simulink model "ROO"  (R2025b)
settings: Solver=VariableStepAuto  StartTime=0.0  StopTime=10  FixedStep=1e-4  RelTol=1e-3
values from neighbouring files (symbols this model uses):
  A_new = T * A * T'    [ROO_code.m]
  Ahat = Abb - Ke * Aab    [ROO_code.m]
  B_new = T * B    [ROO_code.m]
  Bhat = (Abb - Ke*Aab)*Ke + Aba - Ke*Aaa    [ROO_code.m]
  C_new = C * T'    [ROO_code.m]
  Chat = [0 0 0 0 ... (first row only)    [ROO_code.m]
  Dhat = [eye(2);            Ke]    [ROO_code.m]
  eta0_observer = double(xu_start_guess - Ke * y_start_guess)    [ROO_code.m]
  fc = 2 * pi * 15    (= 94.2477796077)    [FSO_code.m]    (also in ROO_code.m)
  Fhat = Bb - Ke * Ba    [ROO_code.m]
  K_new = K * T'    [ROO_code.m]
  params =     [model_data.mat]
  x0_plant = [deg2rad(10); 0; 0; 0; 0; 0]    [ROO_code.m]
libraries: simulink_extras x2, commchan3 x1
settings Model: Creator=Lenovo  LastModifiedBy=Lenovo

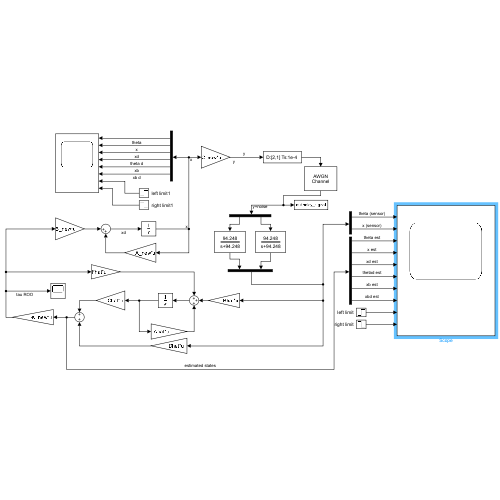
[thumbnail: Simulink's stored preview of the top-level diagram]
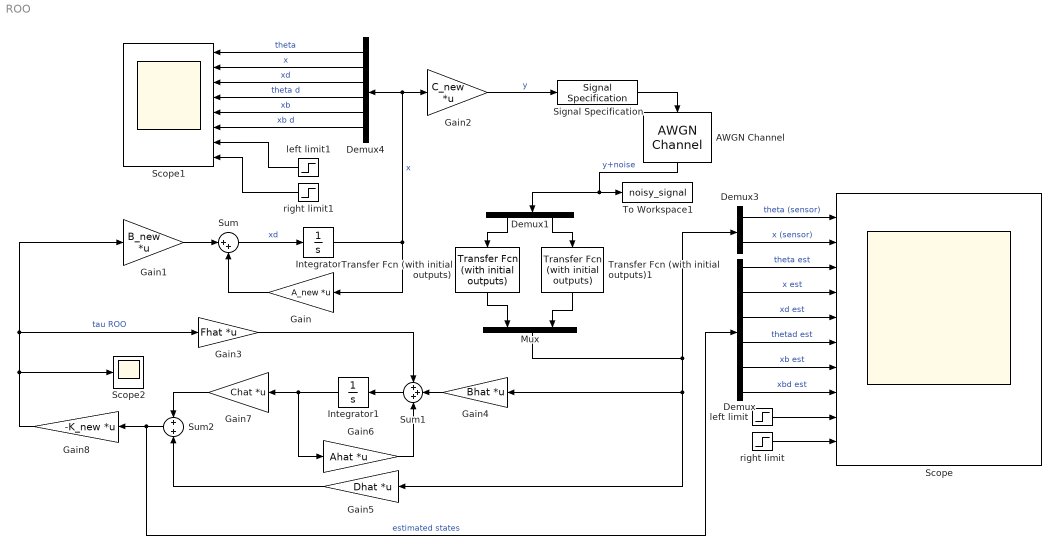
== system ROO ==
  AWGN Channel : commchan3/AWGN Channel  LegacyMode=off  NoiseMethod="Signal to noise ratio  (SNR)"  noiseMode="Signal to noise ratio  (SNR)"  EbNo=10  EsNo=10  SNR=30  BitsPerSymbol=1  SignalPower=1  SpecifySymbolPeriod=off  SamplesPerSymbol=1  SymbolPeriod=1  VarianceSource=Parameter  Variance=1  RandomStream=Global stream  Seed=67  SimulateUsing=Code generation
  Demux : Demux  Outputs=6
  Demux1 : Demux  Outputs=2
  Demux3 : Demux  Outputs=2
  Demux4 : Demux  Outputs=6
  Gain : Gain  Gain=A_new  Multiplication=Matrix(K*u)
  Gain1 : Gain  Gain=B_new  Multiplication=Matrix(K*u)
  Gain2 : Gain  Gain=C_new  Multiplication=Matrix(K*u)
  Gain3 : Gain  Gain=Fhat  Multiplication=Matrix(K*u)
  Gain4 : Gain  Gain=Bhat  Multiplication=Matrix(K*u)
  Gain5 : Gain  Gain=Dhat  Multiplication=Matrix(K*u)
  Gain6 : Gain  Gain=Ahat  Multiplication=Matrix(K*u)
  Gain7 : Gain  Gain=Chat  Multiplication=Matrix(K*u)
  Gain8 : Gain  Gain=-K_new  Multiplication=Matrix(K*u)
  Integrator : Integrator  InitialCondition=x0_plant
  Integrator1 : Integrator  InitialCondition=eta0_observer
  Mux : Mux  Inputs=2
  Scope : Scope  NumInputPorts=10
      settings: SampleTime=1e-4  ActiveDisplayYMinimum=-0.13756249999999998  ActiveDisplayYMaximum=0.13756249999999998
  Scope1 : Scope  NumInputPorts=8
      settings: SampleTime=1e-4  ActiveDisplayYMinimum=-1.4770196744497439  ActiveDisplayYMaximum=11.337524918716566
  Scope2 : Scope
      settings: ActiveDisplayYMinimum=-5.0707763881574976  ActiveDisplayYMaximum=15.205716333962702  DataLoggingVariableName=ScopeData2
  Signal Specification : SignalSpecification  Dimensions=[2,1]  SampleTime=1e-4
  Sum : Sum  Inputs=|++
  Sum1 : Sum  Inputs=+++
  Sum2 : Sum
  To Workspace1 : ToWorkspace  VariableName=noisy_signal  SaveFormat=Structure With Time  SampleTime=1e-4
  Transfer Fcn (with initial outputs) : simulink_extras/Additional Linear/Transfer Fcn (with initial outputs)  N=[fc]  D=[1 fc]  Y0=x0_plant(1)  U0=0
  Transfer Fcn (with initial outputs)1 : simulink_extras/Additional Linear/Transfer Fcn (with initial outputs)  N=[fc]  D=[1 fc]  Y0=x0_plant(2)  U0=0
  left limit : Step  Time=0  After=params.d/2  SampleTime=0
  left limit1 : Step  Time=0  After=params.d/2  SampleTime=0
  right limit : Step  Time=0  After=-params.d/2  SampleTime=0
  right limit1 : Step  Time=0  After=-params.d/2  SampleTime=0
  wires:
  Gain1/1 -> Sum/1
  Gain/1 -> Sum/2
  Gain5/1 -> Sum2/2
  Sum/1 -> Integrator/1  "xd"
  Integrator/1 -> Gain2/1, Demux4/1, Gain/1  "x"
  Gain4/1 -> Sum1/2
  Sum1/1 -> Integrator1/1
  Gain6/1 -> Sum1/3
  Integrator1/1 -> Gain6/1, Gain7/1
  Gain7/1 -> Sum2/1
  Sum2/1 -> Gain8/1, Demux/1  "estimated states"
  Gain8/1 -> Scope2/1, Gain1/1, Gain3/1  "tau ROO"
  left limit/1 -> Scope/9
  right limit/1 -> Scope/10
  Gain3/1 -> Sum1/1
  Demux/5 -> Scope/7  "xb est"
  Demux/6 -> Scope/8  "xbd est"
  Demux/1 -> Scope/3  "theta est"
  Demux/2 -> Scope/4  "x est"
  Demux/3 -> Scope/5  "xd est"
  Demux/4 -> Scope/6  "thetad est"
  Demux3/1 -> Scope/1  "theta (sensor)"
  Demux3/2 -> Scope/2  "x (sensor)"
  Demux4/1 -> Scope1/1  "theta"
  Demux4/2 -> Scope1/2  "x"
  Demux4/3 -> Scope1/3  "xd"
  Demux4/4 -> Scope1/4  "theta d"
  Demux4/5 -> Scope1/5  "xb"
  Demux4/6 -> Scope1/6  "xb d"
  Demux1/1 -> Transfer Fcn (with initial outputs)/1
  Mux/1 -> Gain5/1, Gain4/1, Demux3/1
  right limit1/1 -> Scope1/8
  left limit1/1 -> Scope1/7
  Gain2/1 -> Signal Specification/1  "y"
  Demux1/2 -> Transfer Fcn (with initial outputs)1/1
  AWGN Channel/1 -> Demux1/1, To Workspace1/1  "y+noise"
  Signal Specification/1 -> AWGN Channel/1
  Transfer Fcn (with initial outputs)1/1 -> Mux/2
  Transfer Fcn (with initial outputs)/1 -> Mux/1
